simulink model "FlightController"  (R2023a)
settings: Solver=FixedStepAuto  StartTime=0.0  StopTime=10.0  RelTol=1e-3  EnableMultiTasking=on
undefined symbols (not defined in the file): SampleTime
libraries: matrix_library x1, aerolibutil x1, sharedtransform x1
settings Model: ExtModeTrigDuration=10  Creator=The MathWorks, Inc.  LastModifiedBy=adan
settings SolverCC: AlgebraicLoopSolver=TrustRegion  PositivePriorityOrder=on  MaxZcPerStep=1
settings OptimizationCC: EnhancedBackFolding=on  PassReuseOutputArgsAs=Individual arguments  ZeroExternalMemoryAtStartup=off  ZeroInternalMemoryAtStartup=off  MaxStackSize=64  OptimizeBlockOrder=speed  DifferentSizesBufferReuse=on  OptimizationCustomize=off  EfficientTunableParamExpr=on
settings DebuggingCC: ParameterTunabilityLossMsg=error  UnconnectedInputMsg=warning  UnconnectedOutputMsg=warning  UnconnectedLineMsg=warning
settings HardwareCC: ProdBitPerPointer=32  ProdBitPerSizeT=32  ProdBitPerPtrDiffT=32  ProdLargestAtomicInteger=Long  ProdLargestAtomicFloat=Double  ProdWordSize=32  ProdLongLongMode=on  ProdHWDeviceType=ARM Compatible->ARM Cortex
settings ModelReferenceCC: EnableRefExpFcnMdlSchedulingChecks=on  ModelReferenceNumInstancesAllowed=Single
settings SFSimCC: MATLABDynamicMemAlloc=off  SimTargetLang=C++
settings RTWCC: Description=Embedded Coder  SystemTargetFile=ert.tlc  HardwareBoard=PX4 Host Target  TLCOptions="-aInlineSetEventsForThisBaseRateFcn=TLC_FALSE -aSuppressMultiTaskScheduler=TLC_FALSE  -aRateBasedStepFcn=0"  TemplateMakefile=ert_default_tmf  Toolchain=GNU Tools for PX4 Autopilots  PortableWordSizes=on  TargetLang=C++  DLArmComputeVersion=19.05
settings CodeAppCC: ForceParamTrailComments=on  IgnoreCustomStorageClasses=off  OperatorAnnotations=on  SimulinkDataObjDesc=on  SFDataObjDesc=on  InsertBlockDesc=on
settings ERTTargetCC: ExtModeTransport=2  ExtModeStaticAlloc=on  ExtModeMexFile=ext_xcp  ExtModeIntrfLevel=Level2 - Open

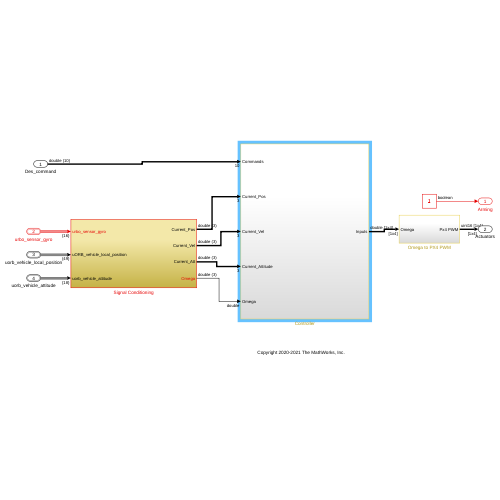
[thumbnail: Simulink's stored preview of the top-level diagram]
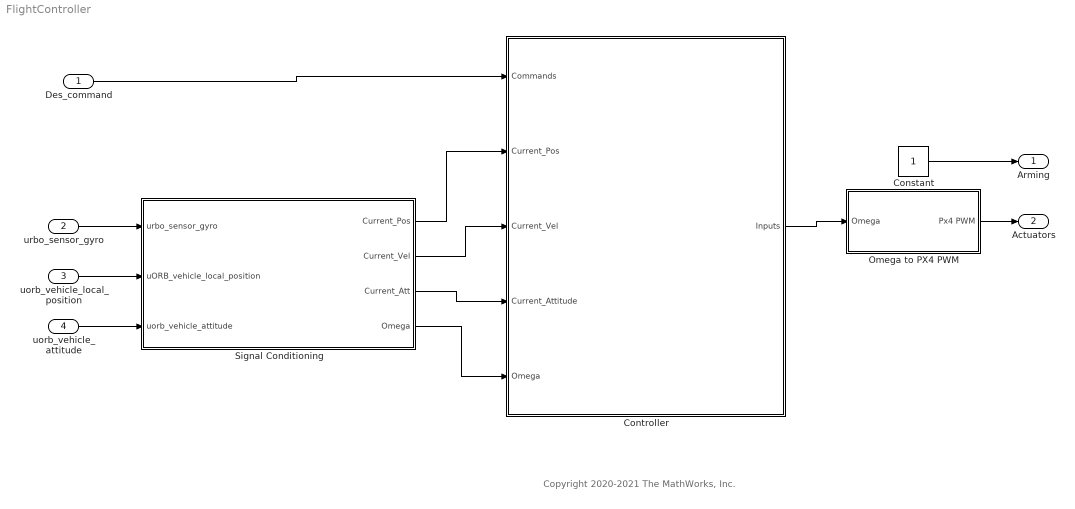
== system FlightController ==
  note: Copyright 2020-2021 The MathWorks, Inc.
  Des_command : Inport
  urbo_sensor_gyro : Inport  Port=2  OutDataTypeStr=Bus: px4_Bus_sensor_gyro
  uorb_vehicle_local_position : Inport  Port=3  OutDataTypeStr=Bus: px4_Bus_vehicle_local_position
  uorb_vehicle_attitude : Inport  Port=4  OutDataTypeStr=Bus: px4_Bus_vehicle_attitude
  Constant : Constant  OutDataTypeStr=boolean  SampleTime=SampleTime
  Controller : Subsystem
  Omega to PX4 PWM : Subsystem
  Signal Conditioning : Subsystem
  Arming : Outport
  Actuators : Outport  Port=2
  wires:
  Constant/1 -> Arming/1
  Omega to PX4 PWM/1(Px4 PWM) -> Actuators/1
  Controller/1(Inputs) -> Omega to PX4 PWM/1(Omega)
  Des_command/1 -> Controller/1(Commands)
  Signal Conditioning/2(Current_Vel) -> Controller/3(Current_Vel)
  uorb_vehicle_local_position/1 -> Signal Conditioning/2(uORB_vehicle_local_position)
  Signal Conditioning/3(Current_Att) -> Controller/4(Current_Attitude)
  uorb_vehicle_attitude/1 -> Signal Conditioning/3(uorb_vehicle_attitude)
  Signal Conditioning/1(Current_Pos) -> Controller/2(Current_Pos)
  urbo_sensor_gyro/1 -> Signal Conditioning/1(urbo_sensor_gyro)
  Signal Conditioning/4(Omega) -> Controller/5(Omega)

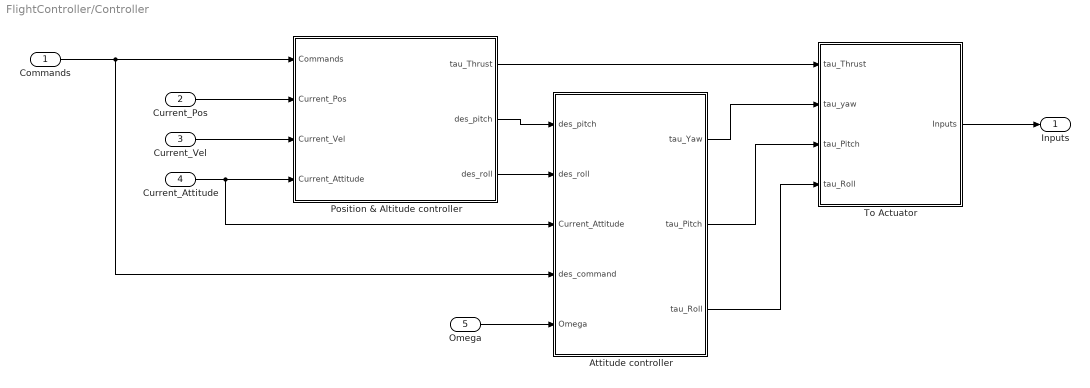
== system FlightController/Controller ==
  Commands : Inport
  Current_Pos : Inport  Port=2
  Current_Vel : Inport  Port=3
  Current_Attitude : Inport  Port=4
  Omega : Inport  Port=5
  Attitude controller : Subsystem
  Position & Altitude controller : Subsystem
  To Actuator : Subsystem
  Inputs : Outport
  wires:
  Current_Attitude/1 -> Attitude controller/3(Current_Attitude), Position & Altitude controller/4(Current_Attitude)
  Position & Altitude controller/3(des_roll) -> Attitude controller/2(des_roll)
  Position & Altitude controller/1(tau_Thrust) -> To Actuator/1(tau_Thrust)
  Attitude controller/1(tau_Yaw) -> To Actuator/2(tau_yaw)
  Attitude controller/3(tau_Roll) -> To Actuator/4(tau_Roll)
  Attitude controller/2(tau_Pitch) -> To Actuator/3(tau_Pitch)
  Position & Altitude controller/2(des_pitch) -> Attitude controller/1(des_pitch)
  Current_Pos/1 -> Position & Altitude controller/2(Current_Pos)
  Current_Vel/1 -> Position & Altitude controller/3(Current_Vel)
  To Actuator/1(Inputs) -> Inputs/1
  Commands/1 -> Attitude controller/4(des_command), Position & Altitude controller/1(Commands)
  Omega/1 -> Attitude controller/5(Omega)

== system FlightController/Omega to PX4 PWM ==
  Omega : Inport
  Constant : Constant  Value=1000  SampleTime=SampleTime
  Data Type Conversion : DataTypeConversion  OutDataTypeStr=uint16  SaturateOnIntegerOverflow=off  RndMeth=Floor
  Gain : Gain  Gain=1000
  Sum : Sum  Inputs=|++
  Px4 PWM : Outport
  wires:
  Data Type Conversion/1 -> Px4 PWM/1
  Sum/1 -> Data Type Conversion/1
  Omega/1 -> Gain/1
  Constant/1 -> Sum/2
  Gain/1 -> Sum/1

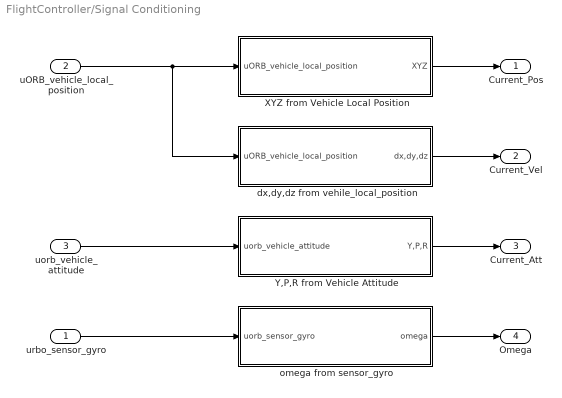
== system FlightController/Signal Conditioning ==
  urbo_sensor_gyro : Inport
  uORB_vehicle_local_position : Inport  Port=2
  uorb_vehicle_attitude : Inport  Port=3
  XYZ from Vehicle Local Position : Subsystem
  Y,P,R from Vehicle Attitude : Subsystem
  dx,dy,dz from vehile_local_position : Subsystem
  omega from sensor_gyro : Subsystem
  Current_Pos : Outport
  Current_Vel : Outport  Port=2
  Current_Att : Outport  Port=3
  Omega : Outport  Port=4
  wires:
  XYZ from Vehicle Local Position/1(XYZ) -> Current_Pos/1
  uORB_vehicle_local_position/1 -> dx,dy,dz from vehile_local_position/1(uORB_vehicle_local_position), XYZ from Vehicle Local Position/1(uORB_vehicle_local_position)
  dx,dy,dz from vehile_local_position/1(dx,dy,dz) -> Current_Vel/1
  uorb_vehicle_attitude/1 -> Y,P,R from Vehicle Attitude/1(uorb_vehicle_attitude)
  Y,P,R from Vehicle Attitude/1(Y,P,R) -> Current_Att/1
  urbo_sensor_gyro/1 -> omega from sensor_gyro/1(uorb_sensor_gyro)
  omega from sensor_gyro/1(omega) -> Omega/1

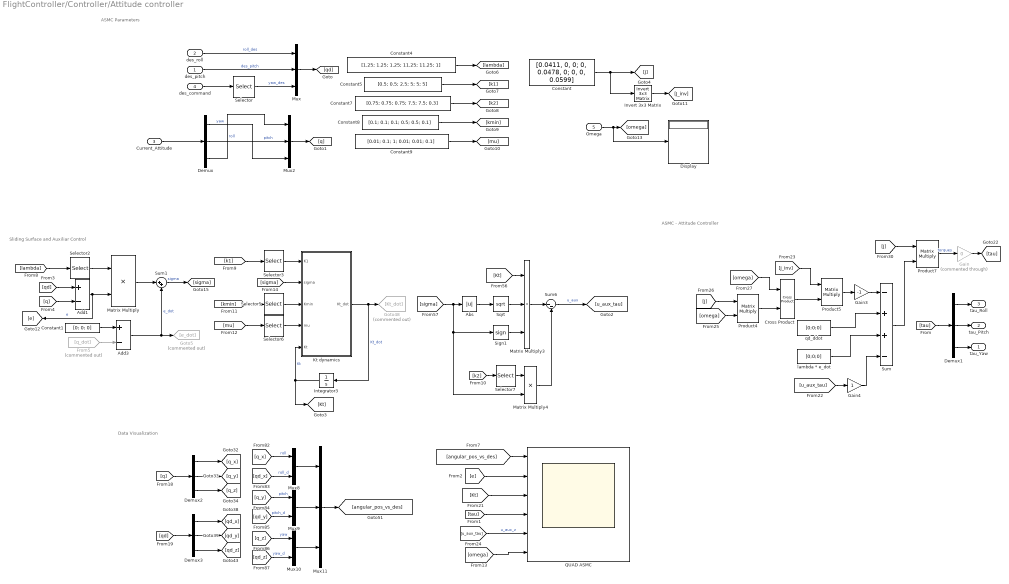
== system FlightController/Controller/Attitude controller ==
  note: Data Visualization
  note: ASMC Parameters
  note: Sliding Surface and Auxiliar Control
  note: ASMC - Attitude Controller
  des_pitch : Inport
  des_roll : Inport  Port=2
  Current_Attitude : Inport  Port=3
  des_command : Inport  Port=4
  Omega : Inport  Port=5
  Abs : Abs  SaturateOnIntegerOverflow=off
  Add1 : Sum  Inputs=+-
  Add3 : Sum  Inputs=+-
  Constant : Constant  Value=[0.0411, 0, 0; 0, 0.0478, 0; 0, 0, 0.0599]
  Constant1 : Constant  Value=[0; 0; 0]
  Constant4 : Constant  Value=[1.25; 1.25; 1.25; 11.25; 11.25; 1]
  Constant5 : Constant  Value=[0.5; 0.5; 2.5; 5; 5; 5]
  Constant7 : Constant  Value=[0.75; 0.75; 0.75; 7.5; 7.5; 0.3]
  Constant8 : Constant  Value=[0.1; 0.1; 0.1; 0.5; 0.5; 0.1]
  Constant9 : Constant  Value=[0.01; 0.1; 1; 0.01; 0.01; 0.1]
  Cross Product : matrix_library/Cross Product
  Demux{,1..3} (4 alike) : Demux  Outputs=3
  Display : Display
  From5 : From  Commented=on  GotoTag=q_dot
  Gain : Gain  Commented=through  Gain=0
  Gain3 : Gain  Gain=-1
  Gain4 : Gain
  Goto48 : Goto  Commented=on  GotoTag=Kt_dot
  Goto5 : Goto  Commented=on  GotoTag=e_dot
  Integrator3 : Integrator  InitialCondition=[0; 0; 0]
  Invert 3x3 Matrix : aerolibutil/Invert  3x3 Matrix
  Kt dynamics : Subsystem
  Matrix Multiply : Product
  Matrix Multiply3 : Product  Inputs=3
  Matrix Multiply4 : Product
  Mux : Mux  Inputs=3
  Mux10 : Mux  Inputs=2
  Mux11 : Mux  Inputs=3
  Mux2 : Mux  Inputs=3
  Mux8 : Mux  Inputs=2
  Mux9 : Mux  Inputs=2
  Product4 : Product  Multiplication=Matrix(*)
  Product5 : Product  Multiplication=Matrix(*)
  Product7 : Product  Multiplication=Matrix(*)
  QUAD ASMC : Scope  NumInputPorts=6
  Selector : Selector  InputPortWidth=10  IndexOptions=Index vector (dialog)  Indices=4  OutputSizes=1
  Selector2 : Selector  InputPortWidth=6  IndexOptions=Index vector (dialog)  Indices=[1:3]  OutputSizes=1
  Selector{3,5..7} (4 alike) : Selector  InputPortWidth=6  IndexOptions=Index vector (dialog)  Indices=[4:6]  OutputSizes=1
  Sign1 : Signum
  Sqrt : Sqrt
  Sum : Sum  Inputs=-++-
  Sum1 : Sum  Inputs=|++
  Sum6 : Sum  Inputs=|--
  lambda * e_dot : Constant  Value=[0;0;0]
  qd_ddot : Constant  Value=[0;0;0]
  tau_Yaw : Outport
  tau_Pitch : Outport  Port=2
  tau_Roll : Outport  Port=3
  wires:
  des_roll/1 -> Mux/1  "roll_des"
  des_pitch/1 -> Mux/2  "des_pitch"
  Selector/1 -> Mux/3  "yaw_des"
  Current_Attitude/1 -> Demux/1
  Demux/3 -> Mux2/1  "roll"
  Demux/1 -> Mux2/3  "yaw"
  Demux/2 -> Mux2/2  "pitch"
  [J] -> Product7/1
  qd_ddot/1 -> Sum/2
  [omega] -> Cross Product/1
  Gain4/1 -> Sum/4
  Gain3/1 -> Sum/1
  [omega] -> Product4/2
  Product5/1 -> Gain3/1
  Product7/1 -> Gain/1  "torques"
  Product4/1 -> Cross Product/2
  Sum/1 -> Product7/2
  Cross Product/1 -> Product5/2
  [u_aux_tau] -> Gain4/1
  [J_inv] -> Product5/1
  [J] -> Product4/1
  [tau] -> Demux1/1
  Demux1/3 -> tau_Yaw/1
  Demux1/2 -> tau_Pitch/1
  Demux1/1 -> tau_Roll/1
  Mux/1 -> [qd]
  Mux2/1 -> [q]
  Constant7/1 -> [k2]
  Constant9/1 -> [mu]
  Constant5/1 -> [k1]
  Constant8/1 -> [kmin]
  Constant4/1 -> [lambda]
  Selector2/1 -> Matrix Multiply/1
  [kmin] -> Selector5/1
  Abs/1 -> Sqrt/1
  Sum1/1 -> [sigma]  "sigma"
  Integrator3/1 -> [Kt], Kt dynamics/5(Kt)  "Kt"
  Selector6/1 -> Kt dynamics/4(mu)
  Matrix Multiply4/1 -> Sum6/2
  Sign1/1 -> Matrix Multiply3/3
  Selector7/1 -> Matrix Multiply4/1
  [mu] -> Selector6/1
  Selector5/1 -> Kt dynamics/3(Kmin)
  [sigma] -> Kt dynamics/2(sigma)
  Selector3/1 -> Kt dynamics/1(K1)
  [k1] -> Selector3/1
  [lambda] -> Selector2/1
  Kt dynamics/1(Kt_dot) -> Integrator3/1, Goto48/1  "Kt_dot"
  Add3/1 -> Goto5/1, Sum1/2  "e_dot"
  [k2] -> Selector7/1
  [qd] -> Add1/1
  [Kt] -> Matrix Multiply3/1
  Matrix Multiply/1 -> Sum1/1
  [sigma] -> Matrix Multiply4/2, Sign1/1, Abs/1
  Sqrt/1 -> Matrix Multiply3/2
  Constant1/1 -> Add3/1
  Sum6/1 -> [u_aux_tau]  "u_aux"
  [q] -> Add1/2
  Matrix Multiply3/1 -> Sum6/1
  From5/1 -> Add3/2
  Add1/1 -> [e], Matrix Multiply/2  "e"
  lambda * e_dot/1 -> Sum/3
  Gain/1 -> [tau]
  [omega] -> QUAD ASMC/6
  [angular_pos_vs_des] -> QUAD ASMC/1
  [tau] -> QUAD ASMC/4
  [Kt] -> QUAD ASMC/3
  [e] -> QUAD ASMC/2
  [u_aux_tau] -> QUAD ASMC/5  "u_aux_z"
  [q_z] -> Mux10/1  "yaw"
  Mux11/1 -> [angular_pos_vs_des]
  Mux8/1 -> Mux11/1
  [q_y] -> Mux9/1  "pitch"
  Demux3/3 -> [qd_z]
  [qd_z] -> Mux10/2  "yaw_d"
  [qd] -> Demux3/1
  [qd_x] -> Mux8/2  "roll_d"
  Demux3/1 -> [qd_x]
  Demux3/2 -> [qd_y]
  Demux2/2 -> [q_y]
  Demux2/1 -> [q_x]
  Mux10/1 -> Mux11/3
  Mux9/1 -> Mux11/2
  Demux2/3 -> [q_z]
  [q] -> Demux2/1
  [qd_y] -> Mux9/2  "pitch_d"
  [q_x] -> Mux8/1  "roll"
  Constant/1 -> Invert 3x3 Matrix/1, [J]
  Invert 3x3 Matrix/1 -> [J_inv]
  Omega/1 -> Display/1, [omega]
  des_command/1 -> Selector/1

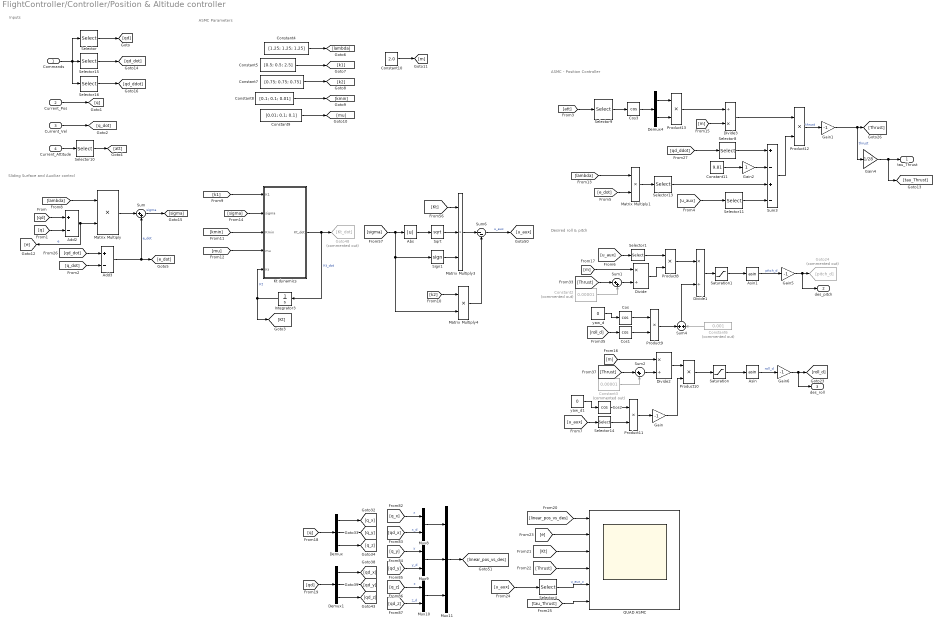
== system FlightController/Controller/Position & Altitude controller ==
  note: Sliding Surface and Auxiliar control
  note: Inputs
  note: ASMC Parameters
  note: ASMC - Position Controller
  note: Desired roll & pitch
  Commands : Inport
  Current_Pos : Inport  Port=2
  Current_Vel : Inport  Port=3
  Current_Attitude : Inport  Port=4
  Abs : Abs  SaturateOnIntegerOverflow=off
  Add2 : Sum  Inputs=+-
  Add3 : Sum  Inputs=+-
  Asin : Trigonometry  Operator=asin
  Asin1 : Trigonometry  Operator=asin
  Constant10 : Constant  Value=2.0
  Constant11 : Constant  Value=9.81
  Constant2 : Constant  Commented=on  Value=0.00001
  Constant3 : Constant  Commented=on  Value=0.00001
  Constant4 : Constant  Value=[1.25; 1.25; 1.25]
  Constant5 : Constant  Value=[0.5; 0.5; 2.5]
  Constant6 : Constant  Commented=on  Value=0.001
  Constant7 : Constant  Value=[0.75; 0.75; 0.75]
  Constant8 : Constant  Value=[0.1; 0.1; 0.01]
  Constant9 : Constant  Value=[0.01; 0.1; 0.1]
  Cos{,1..3} (4 alike) : Trigonometry  Operator=cos
  Demux : Demux  Outputs=3
  Demux1 : Demux  Outputs=3
  Demux4 : Demux  Outputs=2
  Divide : Product  Inputs=*/
  Divide1 : Product  Inputs=*/
  Divide2 : Product  Inputs=*/
  Divide3 : Product  Inputs=/*
  Gain{,1,5..6} (4 alike) : Gain  Gain=-1
  Gain2 : Gain
  Gain4 : Gain  Gain=1/28
  Goto24 : Goto  Commented=on  GotoTag=pitch_d
  Goto48 : Goto  Commented=on  GotoTag=Kt_dot
  Integrator3 : Integrator  InitialCondition=[0; 0; 0]
  Kt dynamics : Subsystem
  Matrix Multiply : Product
  Matrix Multiply1 : Product
  Matrix Multiply3 : Product  Inputs=3
  Matrix Multiply4 : Product
  Mux10 : Mux  Inputs=2
  Mux11 : Mux  Inputs=3
  Mux8 : Mux  Inputs=2
  Mux9 : Mux  Inputs=2
  Product{8..13} (6 alike) : Product
  QUAD ASMC : Scope  NumInputPorts=6
  Saturation : Saturate  UpperLimit=1  LowerLimit=-1
  Saturation1 : Saturate  UpperLimit=1  LowerLimit=-1
  Selector : Selector  InputPortWidth=10  IndexOptions=Index vector (dialog)  Indices=[1:3]  OutputSizes=1
  Selector1 : Selector  InputPortWidth=3  IndexOptions=Index vector (dialog)  Indices=1  OutputSizes=1
  Selector10 : Selector  InputPortWidth=3  IndexOptions=Index vector (dialog)  Indices=[3 2 1]  OutputSizes=1
  Selector{4,8,11,13} (4 alike) : Selector  InputPortWidth=3  IndexOptions=Index vector (dialog)  Indices=3  OutputSizes=1
  Selector14 : Selector  InputPortWidth=3  IndexOptions=Index vector (dialog)  Indices=2  OutputSizes=1
  Selector15 : Selector  InputPortWidth=10  IndexOptions=Index vector (dialog)  Indices=[5:7]  OutputSizes=1
  Selector16 : Selector  InputPortWidth=10  IndexOptions=Index vector (dialog)  Indices=[5:7]  OutputSizes=1
  Selector9 : Selector  InputPortWidth=3  IndexOptions=Index vector (dialog)  Indices=[1 2]  OutputSizes=1
  Sign1 : Signum
  Sqrt : Sqrt
  Sum : Sum  Inputs=|++
  Sum1 : Sum  Inputs=|++
  Sum2 : Sum  Inputs=|++
  Sum3 : Sum  Inputs=+-+-
  Sum4 : Sum
  Sum6 : Sum  Inputs=|--
  yaw_d : Constant  Value=0
  yaw_d1 : Constant  Value=0
  tau_Thrust : Outport
  des_pitch : Outport  Port=2
  des_roll : Outport  Port=3
  wires:
  Current_Pos/1 -> [q]
  [q] -> Add2/2
  [qd] -> Add2/1
  Add2/1 -> [e], Matrix Multiply/2  "e"
  Current_Vel/1 -> [q_dot]
  [qd_dot] -> Add3/1
  Add3/1 -> [e_dot], Sum/2  "e_dot"
  [q_dot] -> Add3/2
  Matrix Multiply/1 -> Sum/1
  Sum/1 -> [sigma]  "sigma"
  Matrix Multiply3/1 -> Sum6/1
  [Kt] -> Matrix Multiply3/1
  Sign1/1 -> Matrix Multiply3/3
  Kt dynamics/1(Kt_dot) -> Integrator3/1, Goto48/1  "Kt_dot"
  Sum6/1 -> [u_aux]  "u_aux"
  Sqrt/1 -> Matrix Multiply3/2
  Abs/1 -> Sqrt/1
  [sigma] -> Matrix Multiply4/2, Sign1/1, Abs/1
  Matrix Multiply4/1 -> Sum6/2
  Integrator3/1 -> [Kt], Kt dynamics/5(Kt)  "Kt"
  [lambda] -> Matrix Multiply/1
  [k1] -> Kt dynamics/1(K1)
  [sigma] -> Kt dynamics/2(sigma)
  [mu] -> Kt dynamics/4(mu)
  [kmin] -> Kt dynamics/3(Kmin)
  [k2] -> Matrix Multiply4/1
  Divide3/1 -> Product12/1
  [att] -> Selector9/1
  Gain1/1 -> Gain4/1, [Thrust]  "thrust"
  Sum3/1 -> Product12/2
  [m] -> Divide3/2
  Demux4/1 -> Product13/1
  Cos3/1 -> Demux4/1
  Gain2/1 -> Sum3/2
  Selector9/1 -> Cos3/1
  [qd_ddot] -> Selector8/1
  Selector11/1 -> Sum3/4
  Constant11/1 -> Gain2/1
  Selector13/1 -> Sum3/3
  Product13/1 -> Divide3/1
  Product12/1 -> Gain1/1  "thrust"
  Selector8/1 -> Sum3/1
  Demux4/2 -> Product13/2
  Current_Attitude/1 -> Selector10/1
  Selector10/1 -> [att]
  [u_aux] -> Selector11/1
  [e_dot] -> Matrix Multiply1/2
  [lambda] -> Matrix Multiply1/1
  Matrix Multiply1/1 -> Selector13/1
  [Thrust] -> Sum1/1
  Asin/1 -> Gain6/1  "roll_d"
  Constant6/1 -> Sum4/2
  Saturation/1 -> Asin/1
  yaw_d/1 -> Cos/1
  Saturation1/1 -> Asin1/1
  Sum4/1 -> Divide1/2
  yaw_d1/1 -> Cos2/1
  Gain6/1 -> des_roll/1, [roll_d]
  Selector1/1 -> Product8/1
  Product9/1 -> Sum4/1
  Sum1/1 -> Divide/2
  Gain/1 -> Product10/2
  Divide2/1 -> Product10/1
  [m] -> Divide2/1
  Constant3/1 -> Sum2/2
  [Thrust] -> Sum2/1
  Constant2/1 -> Sum1/2
  Divide1/1 -> Saturation1/1
  Asin1/1 -> Gain5/1  "pitch_d"
  Selector14/1 -> Product11/2
  Cos2/1 -> Product11/1
  Cos1/1 -> Product9/2
  Product10/1 -> Saturation/1
  Cos/1 -> Product9/1
  Divide/1 -> Product8/2
  [m] -> Divide/1
  [roll_d] -> Cos1/1
  Product8/1 -> Divide1/1
  Product11/1 -> Gain/1
  Gain5/1 -> des_pitch/1, Goto24/1
  Sum2/1 -> Divide2/2
  [u_aux] -> Selector1/1
  [u_aux] -> Selector14/1
  Constant4/1 -> [lambda]
  Constant5/1 -> [k1]
  Constant7/1 -> [k2]
  Constant8/1 -> [kmin]
  Constant9/1 -> [mu]
  Constant10/1 -> [m]
  [q] -> Demux/1
  [qd] -> Demux1/1
  Demux/1 -> [q_x]
  Demux/2 -> [q_y]
  Demux/3 -> [q_z]
  Demux1/2 -> [qd_y]
  Demux1/1 -> [qd_x]
  Demux1/3 -> [qd_z]
  [q_x] -> Mux8/1  "x"
  [qd_x] -> Mux8/2  "x_d"
  Mux9/1 -> Mux11/2
  Mux8/1 -> Mux11/1
  Mux11/1 -> [linear_pos_vs_des]
  [qd_z] -> Mux10/2  "z_d"
  [q_z] -> Mux10/1  "z"
  [qd_y] -> Mux9/2  "y_d"
  [q_y] -> Mux9/1  "y"
  Mux10/1 -> Mux11/3
  [linear_pos_vs_des] -> QUAD ASMC/1
  [e] -> QUAD ASMC/2
  [Kt] -> QUAD ASMC/3
  [Thrust] -> QUAD ASMC/4
  Selector4/1 -> QUAD ASMC/5  "u_aux_z"
  [u_aux] -> Selector4/1
  Gain4/1 -> [tau_Thrust], tau_Thrust/1
  [tau_Thrust] -> QUAD ASMC/6
  Commands/1 -> Selector/1, Selector15/1, Selector16/1
  Selector/1 -> [qd]
  Selector15/1 -> [qd_dot]
  Selector16/1 -> [qd_ddot]

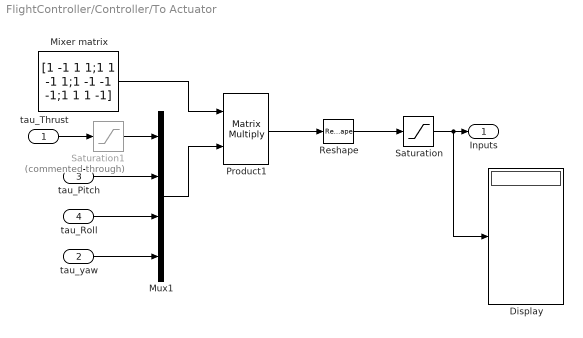
== system FlightController/Controller/To Actuator ==
  tau_Thrust : Inport
  tau_yaw : Inport  Port=2
  tau_Pitch : Inport  Port=3
  tau_Roll : Inport  Port=4
  Display : Display
  Mixer matrix : Constant  Value=[1 -1 1 1;1 1 -1 1;1 -1 -1 -1;1 1 1 -1]  OutDataTypeStr=Inherit: Inherit via back propagation
  Mux1 : Mux
  Product1 : Product  Multiplication=Matrix(*)  RndMeth=Zero
  Reshape : Reshape  OutputDimensionality=Row vector (2-D)
  Saturation : Saturate  UpperLimit=1  LowerLimit=0
  Saturation1 : Saturate  Commented=through  UpperLimit=4*7  LowerLimit=0
  Inputs : Outport
  wires:
  Mixer matrix/1 -> Product1/1
  Mux1/1 -> Product1/2
  tau_Thrust/1 -> Saturation1/1
  Product1/1 -> Reshape/1
  Saturation/1 -> Display/1, Inputs/1
  tau_Pitch/1 -> Mux1/2
  tau_Roll/1 -> Mux1/3
  tau_yaw/1 -> Mux1/4
  Reshape/1 -> Saturation/1
  Saturation1/1 -> Mux1/1

== system FlightController/Signal Conditioning/XYZ from Vehicle Local Position ==
  uORB_vehicle_local_position : Inport
  Bus Selector3 : BusSelector  OutputSignals=x,y,z  OutputAsBus=on
  Data Type Conversion : DataTypeConversion  OutDataTypeStr=double  SaturateOnIntegerOverflow=off  RndMeth=Floor
  XYZ : Outport
  wires:
  uORB_vehicle_local_position/1 -> Bus Selector3/1
  Bus Selector3/1 -> Data Type Conversion/1
  Data Type Conversion/1 -> XYZ/1

== system FlightController/Signal Conditioning/Y,P,R from Vehicle Attitude ==
  uorb_vehicle_attitude : Inport
  Bus Selector2 : BusSelector  OutputSignals=q
  Data Type Conversion1 : DataTypeConversion  OutDataTypeStr=double  SaturateOnIntegerOverflow=off  RndMeth=Floor
  Quaternions to Rotation Angles : sharedtransform/Quaternions to Rotation Angles  rotationOrder=ZYX  aMode=aMode
  Y,P,R : Outport
  wires:
  Bus Selector2/1 -> Data Type Conversion1/1  "<q>"
  Data Type Conversion1/1 -> Quaternions to Rotation Angles/1
  uorb_vehicle_attitude/1 -> Bus Selector2/1
  Quaternions to Rotation Angles/1 -> Y,P,R/1

== system FlightController/Signal Conditioning/dx,dy,dz from vehile_local_position ==
  uORB_vehicle_local_position : Inport
  Bus Selector : BusSelector  OutputSignals=vx,vy,vz  OutputAsBus=on
  Data Type Conversion : DataTypeConversion  OutDataTypeStr=double  SaturateOnIntegerOverflow=off  RndMeth=Floor
  dx,dy,dz : Outport
  wires:
  Bus Selector/1 -> Data Type Conversion/1
  Data Type Conversion/1 -> dx,dy,dz/1
  uORB_vehicle_local_position/1 -> Bus Selector/1

== system FlightController/Signal Conditioning/omega from sensor_gyro ==
  uorb_sensor_gyro : Inport
  Bus Selector3 : BusSelector  OutputSignals=x,y,z  OutputAsBus=on
  Data Type Conversion : DataTypeConversion  OutDataTypeStr=double  SaturateOnIntegerOverflow=off  RndMeth=Floor
  omega : Outport
  wires:
  uorb_sensor_gyro/1 -> Bus Selector3/1
  Bus Selector3/1 -> Data Type Conversion/1
  Data Type Conversion/1 -> omega/1

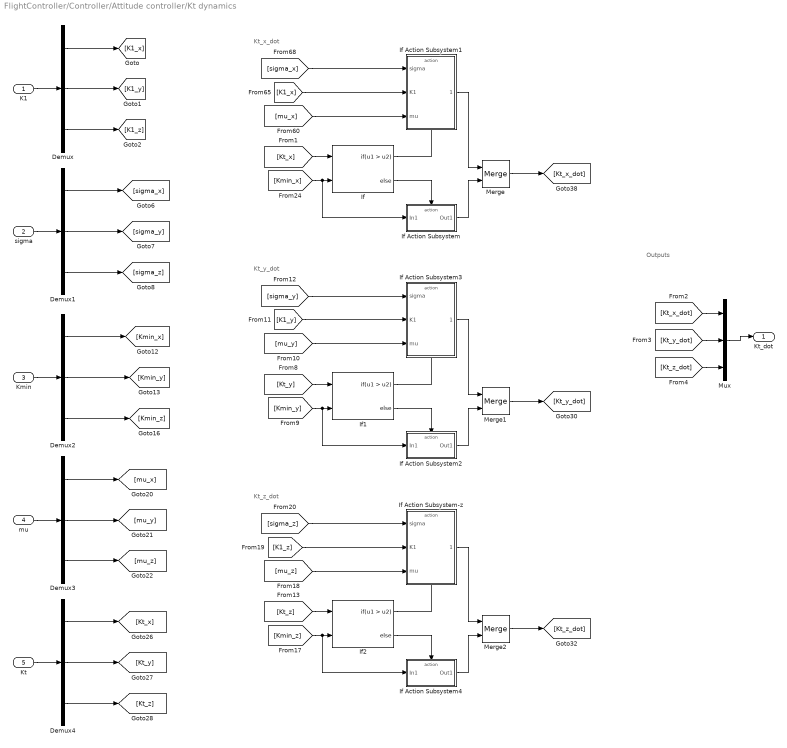
== system FlightController/Controller/Attitude controller/Kt dynamics ==
  note: Outputs
  note: Kt_x_dot
  note: Kt_y_dot
  note: Kt_z_dot
  K1 : Inport
  sigma : Inport  Port=2
  Kmin : Inport  Port=3
  mu : Inport  Port=4
  Kt : Inport  Port=5
  Demux{,1..4} (5 alike) : Demux  Outputs=3
  If : If  NumInputs=2  IfExpression=u1 > u2
  If Action Subsystem : Subsystem  TreatAsAtomicUnit=on
  If Action Subsystem-z : Subsystem  TreatAsAtomicUnit=on
  If Action Subsystem1 : Subsystem  TreatAsAtomicUnit=on
  If Action Subsystem2 : Subsystem  TreatAsAtomicUnit=on
  If Action Subsystem3 : Subsystem  TreatAsAtomicUnit=on
  If Action Subsystem4 : Subsystem  TreatAsAtomicUnit=on
  If1 : If  NumInputs=2  IfExpression=u1 > u2
  If2 : If  NumInputs=2  IfExpression=u1 > u2
  Merge : Merge
  Merge1 : Merge
  Merge2 : Merge
  Mux : Mux  Inputs=3
  Kt_dot : Outport
  wires:
  [Kt_x] -> If/1
  [sigma_x] -> If Action Subsystem1/1(sigma)
  If/1 -> If Action Subsystem1/Action
  [K1_x] -> If Action Subsystem1/2(K1)
  If Action Subsystem1/1(Kt_x_dot) -> Merge/1
  If Action Subsystem/1(Out1) -> Merge/2
  If/2 -> If Action Subsystem/Action
  Merge/1 -> [Kt_x_dot]
  [Kmin_x] -> If Action Subsystem/1(In1), If/2
  [mu_x] -> If Action Subsystem1/3(mu)
  Merge1/1 -> [Kt_y_dot]
  If1/2 -> If Action Subsystem2/Action
  If Action Subsystem2/1(Out1) -> Merge1/2
  If Action Subsystem3/1(Kt_x_dot) -> Merge1/1
  [Kt_y] -> If1/1
  [K1_y] -> If Action Subsystem3/2(K1)
  [mu_y] -> If Action Subsystem3/3(mu)
  [Kmin_y] -> If Action Subsystem2/1(In1), If1/2
  [sigma_y] -> If Action Subsystem3/1(sigma)
  Merge2/1 -> [Kt_z_dot]
  If Action Subsystem-z/1(Kt_z_dot) -> Merge2/1
  [sigma_z] -> If Action Subsystem-z/1(sigma)
  [Kt_z] -> If2/1
  [mu_z] -> If Action Subsystem-z/3(mu)
  [Kmin_z] -> If Action Subsystem4/1(In1), If2/2
  If2/2 -> If Action Subsystem4/Action
  If2/1 -> If Action Subsystem-z/Action
  If Action Subsystem4/1(Out1) -> Merge2/2
  [K1_z] -> If Action Subsystem-z/2(K1)
  If1/1 -> If Action Subsystem3/Action
  Demux4/1 -> [Kt_x]
  Demux1/3 -> [sigma_z]
  Demux1/1 -> [sigma_x]
  Demux1/2 -> [sigma_y]
  Kt/1 -> Demux4/1
  sigma/1 -> Demux1/1
  Demux3/1 -> [mu_x]
  Demux2/3 -> [Kmin_z]
  Demux3/3 -> [mu_z]
  mu/1 -> Demux3/1
  Demux3/2 -> [mu_y]
  Demux2/1 -> [Kmin_x]
  Demux2/2 -> [Kmin_y]
  Demux4/2 -> [Kt_y]
  Demux4/3 -> [Kt_z]
  Demux/1 -> [K1_x]
  K1/1 -> Demux/1
  Demux/2 -> [K1_y]
  Kmin/1 -> Demux2/1
  Demux/3 -> [K1_z]
  Mux/1 -> Kt_dot/1
  [Kt_z_dot] -> Mux/3
  [Kt_x_dot] -> Mux/1
  [Kt_y_dot] -> Mux/2

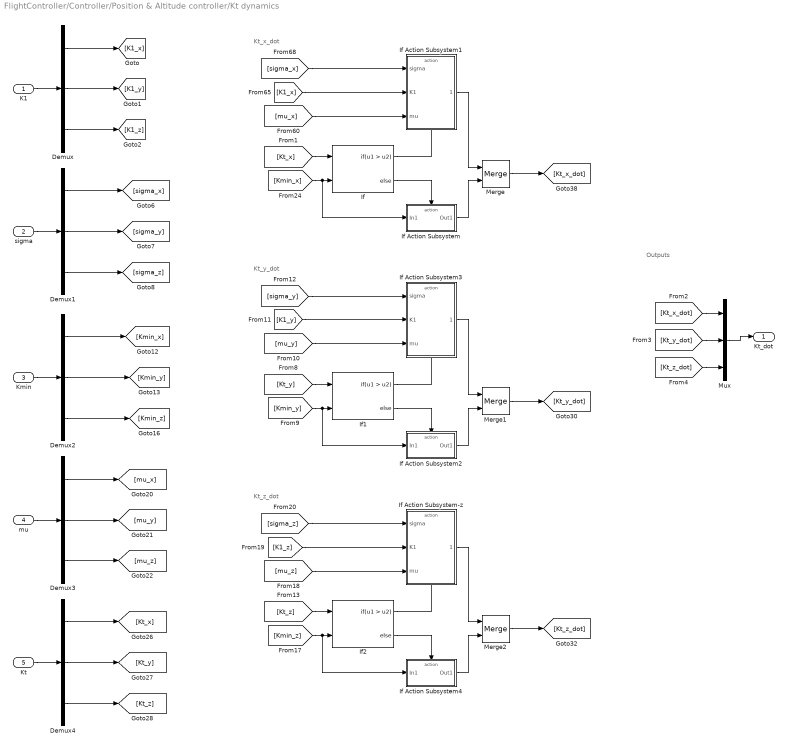
== system FlightController/Controller/Position & Altitude controller/Kt dynamics ==
  note: Outputs
  note: Kt_x_dot
  note: Kt_y_dot
  note: Kt_z_dot
  K1 : Inport
  sigma : Inport  Port=2
  Kmin : Inport  Port=3
  mu : Inport  Port=4
  Kt : Inport  Port=5
  Demux{,1..4} (5 alike) : Demux  Outputs=3
  If : If  NumInputs=2  IfExpression=u1 > u2
  If Action Subsystem : Subsystem  TreatAsAtomicUnit=on
  If Action Subsystem-z : Subsystem  TreatAsAtomicUnit=on
  If Action Subsystem1 : Subsystem  TreatAsAtomicUnit=on
  If Action Subsystem2 : Subsystem  TreatAsAtomicUnit=on
  If Action Subsystem3 : Subsystem  TreatAsAtomicUnit=on
  If Action Subsystem4 : Subsystem  TreatAsAtomicUnit=on
  If1 : If  NumInputs=2  IfExpression=u1 > u2
  If2 : If  NumInputs=2  IfExpression=u1 > u2
  Merge : Merge
  Merge1 : Merge
  Merge2 : Merge
  Mux : Mux  Inputs=3
  Kt_dot : Outport
  wires:
  [Kt_x] -> If/1
  [sigma_x] -> If Action Subsystem1/1(sigma)
  If/1 -> If Action Subsystem1/Action
  [K1_x] -> If Action Subsystem1/2(K1)
  If Action Subsystem1/1(Kt_x_dot) -> Merge/1
  If Action Subsystem/1(Out1) -> Merge/2
  If/2 -> If Action Subsystem/Action
  Merge/1 -> [Kt_x_dot]
  [Kmin_x] -> If Action Subsystem/1(In1), If/2
  [mu_x] -> If Action Subsystem1/3(mu)
  Merge1/1 -> [Kt_y_dot]
  If1/2 -> If Action Subsystem2/Action
  If Action Subsystem2/1(Out1) -> Merge1/2
  If Action Subsystem3/1(Kt_x_dot) -> Merge1/1
  [Kt_y] -> If1/1
  [K1_y] -> If Action Subsystem3/2(K1)
  [mu_y] -> If Action Subsystem3/3(mu)
  [Kmin_y] -> If Action Subsystem2/1(In1), If1/2
  [sigma_y] -> If Action Subsystem3/1(sigma)
  Merge2/1 -> [Kt_z_dot]
  If Action Subsystem-z/1(Kt_z_dot) -> Merge2/1
  [sigma_z] -> If Action Subsystem-z/1(sigma)
  [Kt_z] -> If2/1
  [mu_z] -> If Action Subsystem-z/3(mu)
  [Kmin_z] -> If Action Subsystem4/1(In1), If2/2
  If2/2 -> If Action Subsystem4/Action
  If2/1 -> If Action Subsystem-z/Action
  If Action Subsystem4/1(Out1) -> Merge2/2
  [K1_z] -> If Action Subsystem-z/2(K1)
  If1/1 -> If Action Subsystem3/Action
  Demux4/1 -> [Kt_x]
  Demux1/3 -> [sigma_z]
  Demux1/1 -> [sigma_x]
  Demux1/2 -> [sigma_y]
  Kt/1 -> Demux4/1
  sigma/1 -> Demux1/1
  Demux3/1 -> [mu_x]
  Demux2/3 -> [Kmin_z]
  Demux3/3 -> [mu_z]
  mu/1 -> Demux3/1
  Demux3/2 -> [mu_y]
  Demux2/1 -> [Kmin_x]
  Demux2/2 -> [Kmin_y]
  Demux4/2 -> [Kt_y]
  Demux4/3 -> [Kt_z]
  Demux/1 -> [K1_x]
  K1/1 -> Demux/1
  Demux/2 -> [K1_y]
  Kmin/1 -> Demux2/1
  Demux/3 -> [K1_z]
  Mux/1 -> Kt_dot/1
  [Kt_z_dot] -> Mux/3
  [Kt_x_dot] -> Mux/1
  [Kt_y_dot] -> Mux/2

== system FlightController/Controller/Attitude controller/Kt dynamics/If Action Subsystem ==
  In1 : Inport
  Action Port : ActionPort  ActionPortLabel=else
  Out1 : Outport
  wires:
  In1/1 -> Out1/1

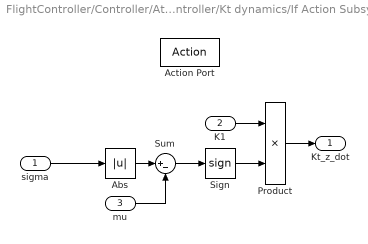
== system FlightController/Controller/Attitude controller/Kt dynamics/If Action Subsystem-z ==
  sigma : Inport
  K1 : Inport  Port=2
  mu : Inport  Port=3
  Action Port : ActionPort  ActionPortLabel=if(u1 > u2)
  Abs : Abs  SaturateOnIntegerOverflow=off
  Product : Product
  Sign : Signum
  Sum : Sum  Inputs=|+-
  Kt_z_dot : Outport
  wires:
  sigma/1 -> Abs/1
  Abs/1 -> Sum/1
  mu/1 -> Sum/2
  Sum/1 -> Sign/1
  Product/1 -> Kt_z_dot/1
  Sign/1 -> Product/2
  K1/1 -> Product/1

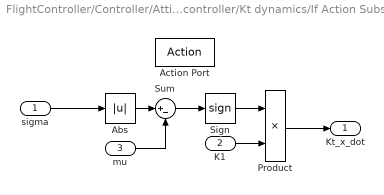
== system FlightController/Controller/Attitude controller/Kt dynamics/If Action Subsystem1 ==
  sigma : Inport
  K1 : Inport  Port=2
  mu : Inport  Port=3
  Action Port : ActionPort  ActionPortLabel=if(u1 > u2)
  Abs : Abs  SaturateOnIntegerOverflow=off
  Product : Product
  Sign : Signum
  Sum : Sum  Inputs=|+-
  Kt_x_dot : Outport
  wires:
  sigma/1 -> Abs/1
  Abs/1 -> Sum/1
  mu/1 -> Sum/2
  Sum/1 -> Sign/1
  Sign/1 -> Product/1
  K1/1 -> Product/2
  Product/1 -> Kt_x_dot/1

== system FlightController/Controller/Attitude controller/Kt dynamics/If Action Subsystem2 ==
  In1 : Inport
  Action Port : ActionPort  ActionPortLabel=else
  Out1 : Outport
  wires:
  In1/1 -> Out1/1

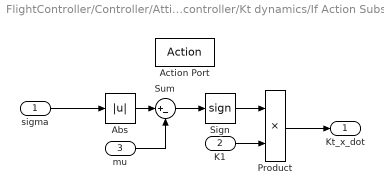
== system FlightController/Controller/Attitude controller/Kt dynamics/If Action Subsystem3 ==
  sigma : Inport
  K1 : Inport  Port=2
  mu : Inport  Port=3
  Action Port : ActionPort  ActionPortLabel=if(u1 > u2)
  Abs : Abs  SaturateOnIntegerOverflow=off
  Product : Product
  Sign : Signum
  Sum : Sum  Inputs=|+-
  Kt_x_dot : Outport
  wires:
  sigma/1 -> Abs/1
  Abs/1 -> Sum/1
  mu/1 -> Sum/2
  Sum/1 -> Sign/1
  Sign/1 -> Product/1
  K1/1 -> Product/2
  Product/1 -> Kt_x_dot/1

== system FlightController/Controller/Attitude controller/Kt dynamics/If Action Subsystem4 ==
  In1 : Inport
  Action Port : ActionPort  ActionPortLabel=else
  Out1 : Outport
  wires:
  In1/1 -> Out1/1

== system FlightController/Controller/Position & Altitude controller/Kt dynamics/If Action Subsystem ==
  In1 : Inport
  Action Port : ActionPort  ActionPortLabel=else
  Out1 : Outport
  wires:
  In1/1 -> Out1/1

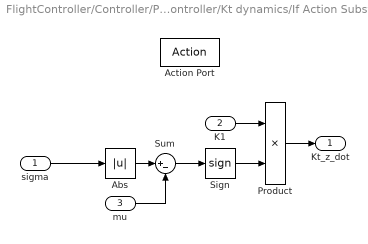
== system FlightController/Controller/Position & Altitude controller/Kt dynamics/If Action Subsystem-z ==
  sigma : Inport
  K1 : Inport  Port=2
  mu : Inport  Port=3
  Action Port : ActionPort  ActionPortLabel=if(u1 > u2)
  Abs : Abs  SaturateOnIntegerOverflow=off
  Product : Product
  Sign : Signum
  Sum : Sum  Inputs=|+-
  Kt_z_dot : Outport
  wires:
  sigma/1 -> Abs/1
  Abs/1 -> Sum/1
  mu/1 -> Sum/2
  Sum/1 -> Sign/1
  Product/1 -> Kt_z_dot/1
  Sign/1 -> Product/2
  K1/1 -> Product/1

== system FlightController/Controller/Position & Altitude controller/Kt dynamics/If Action Subsystem1 ==
  sigma : Inport
  K1 : Inport  Port=2
  mu : Inport  Port=3
  Action Port : ActionPort  ActionPortLabel=if(u1 > u2)
  Abs : Abs  SaturateOnIntegerOverflow=off
  Product : Product
  Sign : Signum
  Sum : Sum  Inputs=|+-
  Kt_x_dot : Outport
  wires:
  sigma/1 -> Abs/1
  Abs/1 -> Sum/1
  mu/1 -> Sum/2
  Sum/1 -> Sign/1
  Sign/1 -> Product/1
  K1/1 -> Product/2
  Product/1 -> Kt_x_dot/1

== system FlightController/Controller/Position & Altitude controller/Kt dynamics/If Action Subsystem2 ==
  In1 : Inport
  Action Port : ActionPort  ActionPortLabel=else
  Out1 : Outport
  wires:
  In1/1 -> Out1/1

== system FlightController/Controller/Position & Altitude controller/Kt dynamics/If Action Subsystem3 ==
  sigma : Inport
  K1 : Inport  Port=2
  mu : Inport  Port=3
  Action Port : ActionPort  ActionPortLabel=if(u1 > u2)
  Abs : Abs  SaturateOnIntegerOverflow=off
  Product : Product
  Sign : Signum
  Sum : Sum  Inputs=|+-
  Kt_x_dot : Outport
  wires:
  sigma/1 -> Abs/1
  Abs/1 -> Sum/1
  mu/1 -> Sum/2
  Sum/1 -> Sign/1
  Sign/1 -> Product/1
  K1/1 -> Product/2
  Product/1 -> Kt_x_dot/1

== system FlightController/Controller/Position & Altitude controller/Kt dynamics/If Action Subsystem4 ==
  In1 : Inport
  Action Port : ActionPort  ActionPortLabel=else
  Out1 : Outport
  wires:
  In1/1 -> Out1/1
